simulink model "T1_PreLab_1"  (R2023a)
settings: Solver=VariableStepAuto  StartTime=0.0  StopTime=3  RelTol=1e-3
libraries: dspfdesign x3, dspmathops x2, dspsrcs4 x1
settings Model: Creator=HP VICTUS  LastModifiedBy=HP VICTUS

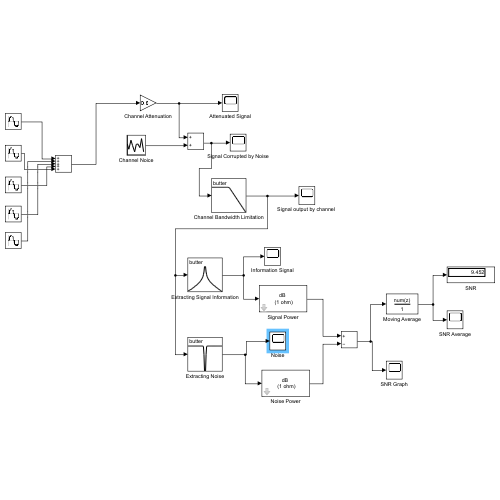
[thumbnail: Simulink's stored preview of the top-level diagram]
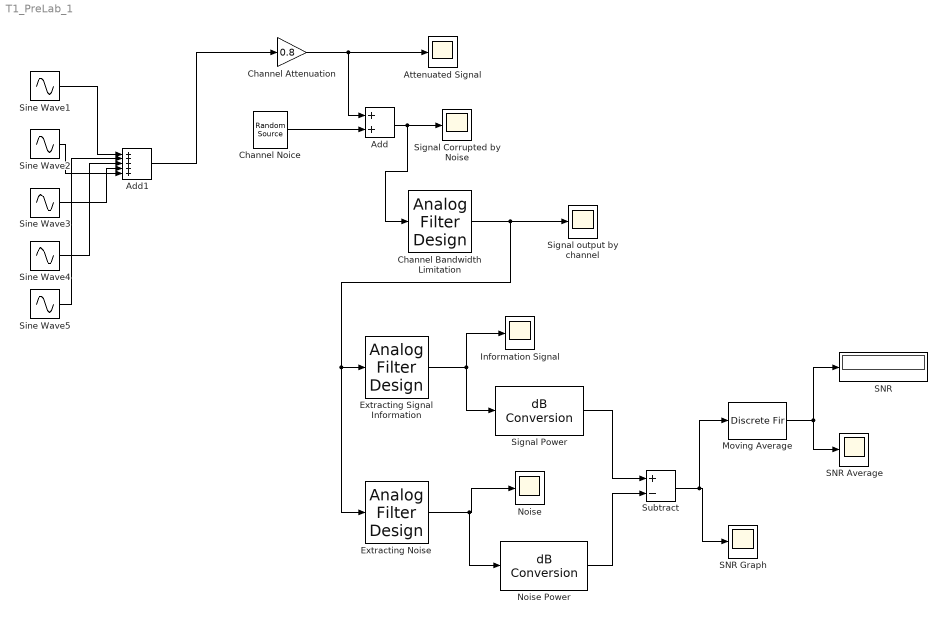
== system T1_PreLab_1 ==
  Add : Sum
  Add1 : Sum  Inputs=+++++
  Attenuated Signal : Scope
  Channel Attenuation : Gain  Gain=0.8
  Channel Bandwidth Limitation : dspfdesign/Analog Filter Design  method=Butterworth  filttype=Lowpass  N=10  Wlo=1000  Whi=80  Rp=2  Rs=40
  Channel Noice : dspsrcs4/Random Source  SrcType=Gaussian  NormMethod=Ziggurat  CltLength=12  MinVal=0  MaxVal=1  MeanVal=0  VarVal=2  RepMode=Not repeatable  rawSeed=1  IsInherit=off  SampMode=Discrete  SampTime=0.001  SampFrame=1  DataType=Double  OutComplex=Real  OutputFrames=off
  Extracting Noise : dspfdesign/Analog Filter Design  method=Butterworth  filttype=Bandstop  N=10  Wlo=195  Whi=285  Rp=2  Rs=40
  Extracting Signal Information : dspfdesign/Analog Filter Design  method=Butterworth  filttype=Bandpass  N=10  Wlo=195  Whi=205  Rp=2  Rs=40
  Information Signal : Scope
  Moving Average : DiscreteFir  Coefficients=ones(1,1000)/1000  SampleTime=0.001
  Noise : Scope
  Noise Power : dspmathops/dB Conversion  dBtype=dB  intype=Amplitude  R=1  fuzz=off
      settings: LibrarySourceBlock=commutil2/dB Conversion
  SNR : Display
  SNR Average : Scope
  SNR Graph : Scope
  Signal Corrupted by Noise : Scope
  Signal Power : dspmathops/dB Conversion  dBtype=dB  intype=Amplitude  R=1  fuzz=off
      settings: LibrarySourceBlock=commutil2/dB Conversion
  "Signal output by channel " : Scope
  Sine Wave1 : Sin  Amplitude=10  Frequency=200  SampleTime=0.001
  Sine Wave2 : Sin  Amplitude=8  Frequency=220  SampleTime=0.001
  Sine Wave3 : Sin  Amplitude=6  Frequency=240  SampleTime=0.001
  Sine Wave4 : Sin  Amplitude=4  Frequency=260  SampleTime=0.001
  Sine Wave5 : Sin  Amplitude=2  Frequency=280  SampleTime=0.001
  Subtract : Sum  Inputs=+-
  wires:
  Channel Attenuation/1 -> Add/1, Attenuated Signal/1
  Channel Noice/1 -> Add/2
  Add/1 -> Channel Bandwidth Limitation/1, Signal Corrupted by Noise/1
  Channel Bandwidth Limitation/1 -> Extracting Signal Information/1, Extracting Noise/1, "Signal output by channel "/1
  Extracting Signal Information/1 -> Signal Power/1, Information Signal/1
  Extracting Noise/1 -> Noise Power/1, Noise/1
  Signal Power/1 -> Subtract/1
  Noise Power/1 -> Subtract/2
  Subtract/1 -> Moving Average/1, SNR Graph/1
  Moving Average/1 -> SNR Average/1, SNR/1
  Sine Wave1/1 -> Add1/1
  Sine Wave2/1 -> Add1/5
  Sine Wave3/1 -> Add1/4
  Sine Wave4/1 -> Add1/3
  Sine Wave5/1 -> Add1/2
  Add1/1 -> Channel Attenuation/1
